simulink model "Kugelanschliff"  (Simulink 6.2)
settings: Solver=ode23s  StartTime=0.0  StopTime=7  FixedStep=0.01  RelTol=1e-3
values from neighbouring files (symbols this model uses):
  a = (2*r*pi)/(kp*vs)    (= 31415926.5359)    [Anschleifen_Init.m]
  b = pi/(kp*vs)    (= 1570796326.79)    [Anschleifen_Init.m]
  kf = 1/((1/c1)+(1/c2))    [Anschleifen_Init.m]
  kp = 0.2e-9    (= 2e-10)    [Anschleifen_Init.m]
  my = 0.2    [Anschleifen_Init.m]
  r = 10e-3    (= 0.01)    [Anschleifen_Init.m]
  vs = 10    [Anschleifen_Init.m]
  vz = 2e-3    (= 0.002)    [Anschleifen_Init.m]
libraries: simulink x1
settings Model: LastModifiedBy=Frowald
settings SolverCC: InitialStep=0.00001  SolverResetMethod=Robust
settings DebuggingCC: SolverPrmCheckMsg=warning

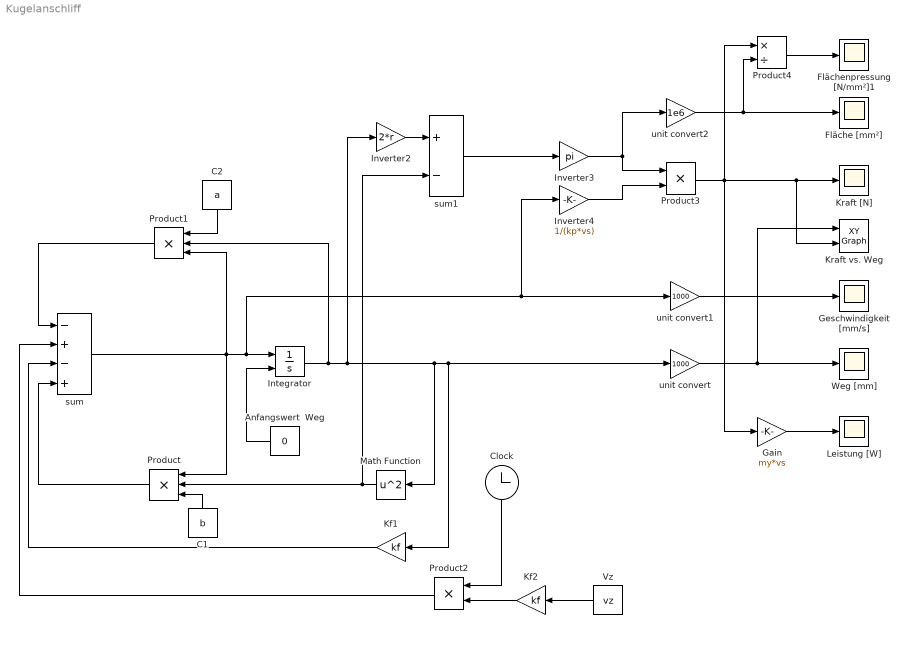
== system Kugelanschliff ==
  Anfangswert  Weg : Constant  Orientation=left  Value=0
  C1 : Constant  Orientation=up  Value=b
  C2 : Constant  Orientation=down  Value=a
  Clock : Clock
      settings: Orientation=down  Decimation=10
  Fläche [mm²] : Scope
      settings: TimeRange=7  YMin=-2.015  YMax=-1.96  SaveName=ScopeData3
  Flächenpressung [N/mm²]1 : Scope
      settings: TimeRange=7  YMin=-2.015  YMax=-1.96  SaveName=ScopeData4
  Gain : Gain  Gain=my*vs
  Geschwindigkeit [mm/s] : Scope
      settings: TimeRange=7  YMin=-2.015  YMax=-1.96
  Integrator : Integrator  InitialConditionSource=external  InitialCondition=-2*10^-3
  Inverter2 : Gain  Gain=2*r
  Inverter3 : Gain  Gain=pi
  Inverter4 : Gain  Gain=1/(kp*vs)
  Kf1 : Gain  Orientation=left  Gain=kf
  Kf2 : Gain  Orientation=left  Gain=kf
  Kraft [N] : Scope
      settings: TimeRange=7  YMin=-2.015  YMax=-1.96  SaveName=ScopeData2
  Kraft vs. Weg : simulink/Sinks/XY Graph  xmin=0  xmax=14  ymin=0  ymax=500  st=-1
  Leistung [W] : Scope
      settings: TimeRange=10  YMin=0  YMax=180  SaveName=ScopeData5
  Math Function : Math  Orientation=left  Operator=square  SaturateOnIntegerOverflow=on
  Product : Product  Orientation=left  Inputs=***  RndMeth=Zero
  Product1 : Product  Orientation=left  Inputs=***  RndMeth=Zero
  Product2 : Product  Orientation=left  Inputs=**  RndMeth=Zero
  Product3 : Product  Inputs=**  RndMeth=Zero
  Product4 : Product  Inputs=*/  RndMeth=Zero
  Vz : Constant  Orientation=left  Value=vz
  Weg [mm] : Scope
      settings: TimeRange=10  YMin=0  YMax=180
  sum : Sum  Inputs=-+-+  OutScaling=2^-10
  sum1 : Sum  Inputs=+-  OutScaling=2^-10
  unit convert : Gain  Gain=1000
  unit convert1 : Gain  Gain=1000
  unit convert2 : Gain  Gain=1e6
  wires:
  C2/1 -> Product1/1
  C1/1 -> Product/3
  Integrator/1 -> Product1/2, Math Function/1, Kf1/1, unit convert/1, Inverter2/1
  sum/1 -> Product1/3, Product/1, Integrator/1, unit convert1/1, Inverter4/1
  Clock/1 -> Product2/1
  Kf1/1 -> sum/3
  Product/1 -> sum/4
  Product2/1 -> sum/2
  Product1/1 -> sum/1
  Math Function/1 -> Product/2, sum1/2
  unit convert1/1 -> Geschwindigkeit [mm/s]/1
  Anfangswert  Weg/1 -> Integrator/2
  unit convert/1 -> Weg [mm]/1, Kraft vs. Weg/1
  Inverter2/1 -> sum1/1
  sum1/1 -> Inverter3/1
  Inverter3/1 -> Product3/1, unit convert2/1
  Inverter4/1 -> Product3/2
  Product3/1 -> Kraft [N]/1, Kraft vs. Weg/2, Gain/1, Product4/1
  unit convert2/1 -> Fläche [mm²]/1, Product4/2
  Vz/1 -> Kf2/1
  Kf2/1 -> Product2/2
  Product4/1 -> Flächenpressung [N/mm²]1/1
  Gain/1 -> Leistung [W]/1
